simulink model "mobrob_sim"  (Simulink 7.2)
settings: Solver=ode45  StartTime=0.0  StopTime=60  FixedStep=0.1*Ts  RelTol=1e-3
values from neighbouring files (symbols this model uses):
  robot = jacobian(robot, q)    [contactforce.m]    (also in dirkin.m = robotIn; dyn.m = dynmodel2(robot,q,dq,Ftool); dynmodel.m = neinit(robotIn,q); dynmodel2.m = neinit(robotIn,q))
  x0 = 0    [RV_EKF_sim.m]    (also in dyn.m = [q0; dq0])
undefined symbols (not defined in the file or in its folder): ctrlparam, map
settings Model: Creator=Cupec  LastModifiedBy=Cupec
settings OptimizationCC: InitFltsAndDblsToZero=on
settings DebuggingCC: SaveWithParameterizedLinksMsg=none  SignalResolutionControl=TryResolveAllWithWarning  MultiTaskDSMMsg=warning  MultiTaskCondExecSysMsg=none
settings RTWCC: IncludeERTFirstTime=on
settings GRTTargetCC: TargetFcnLib=ansi_tfl_tmw.mat

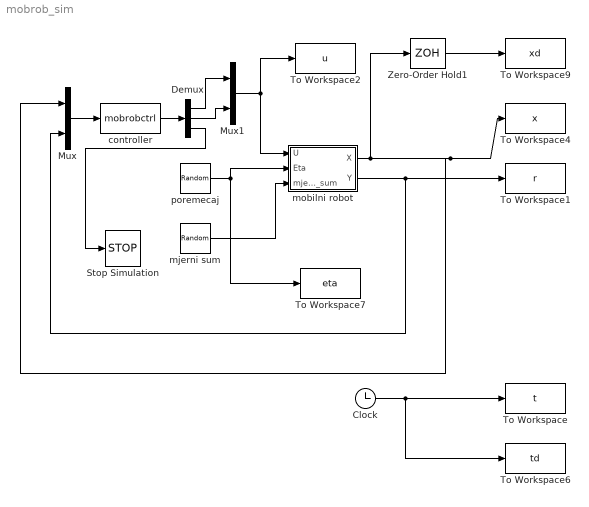
== system mobrob_sim ==
  Clock : Clock
      settings: Decimation=10
  Demux : Demux  Outputs=3
  Mux : Mux  Inputs=2
  Mux1 : Mux  Inputs=2
  Stop Simulation : Stop
  To Workspace : ToWorkspace  VariableName=t  SampleTime=-1  SaveFormat=Array
  To Workspace1 : ToWorkspace  VariableName=r  SampleTime=0.1*robot.TS  SaveFormat=Array
  To Workspace2 : ToWorkspace  VariableName=u  SampleTime=0.1*ctrlparam.T  SaveFormat=Array
  To Workspace4 : ToWorkspace  VariableName=x  SampleTime=-1  SaveFormat=Array
  To Workspace6 : ToWorkspace  VariableName=td  SampleTime=0.1*ctrlparam.T  SaveFormat=Array
  To Workspace7 : ToWorkspace  VariableName=eta  SampleTime=0.1*ctrlparam.T  SaveFormat=Array
  To Workspace9 : ToWorkspace  VariableName=xd  SampleTime=0.1*ctrlparam.T  SaveFormat=Array
  Zero-Order Hold1 : ZeroOrderHold  SampleTime=ctrlparam.T
  controller : S-Function  FunctionName=mobrobctrl  Parameters=robot,ctrlparam,map  EnableBusSupport=off
  mjerni sum : RandomNumber  Mean=zeros(robot.nS,1)  Variance=robot.varnoise*ones(robot.nS,1)  Seed=100100  SampleTime=0.1*ctrlparam.T
  mobilni robot : Subsystem
  poremecaj : RandomNumber  Mean=zeros(2,1)  Variance=robot.vardisturb*ones(2,1)  Seed=[30018 67776]'  SampleTime=0.1*ctrlparam.T
  wires:
  Clock/1 -> To Workspace/1, To Workspace6/1
  mobilni robot/1(X) -> Zero-Order Hold1/1, To Workspace4/1, Mux/1
  poremecaj/1 -> To Workspace7/1, mobilni robot/2(Eta)
  Mux/1 -> controller/1
  Zero-Order Hold1/1 -> To Workspace9/1
  mjerni sum/1 -> mobilni robot/3(mjerni_sum)
  mobilni robot/2(Y) -> To Workspace1/1, Mux/2
  controller/1 -> Demux/1
  Demux/1 -> Mux1/1
  Demux/2 -> Mux1/2
  Mux1/1 -> To Workspace2/1, mobilni robot/1(U)
  Demux/3 -> Stop Simulation/1

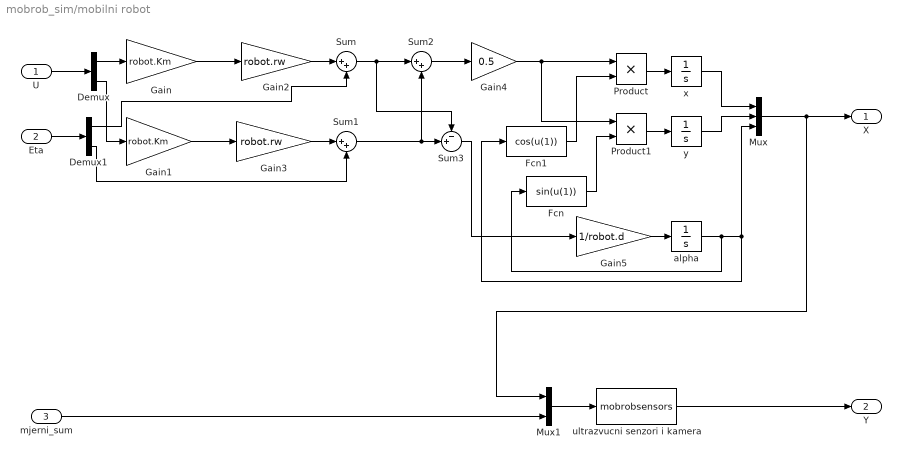
== system mobrob_sim/mobilni robot ==
  U : Inport  OutDataType=sfix(16)  OutScaling=2^0
  Eta : Inport  Port=2  OutDataType=sfix(16)  OutScaling=2^0
  mjerni_sum : Inport  Port=3  OutDataType=sfix(16)  OutScaling=2^0
  Demux : Demux  Outputs=[1 1]
  Demux1 : Demux  Outputs=[1 1]
  Fcn : Fcn  Expr=sin(u(1))
  Fcn1 : Fcn  Expr=cos(u(1))
  Gain : Gain  Gain=robot.Km  ParameterDataType=sfix(16)  ParameterScaling=2^0  OutDataType=sfix(16)  OutScaling=2^0
  Gain1 : Gain  Gain=robot.Km  ParameterDataType=sfix(16)  ParameterScaling=2^0  OutDataType=sfix(16)  OutScaling=2^0
  Gain2 : Gain  Gain=robot.rw  ParameterDataType=sfix(16)  ParameterScaling=2^0  OutDataType=sfix(16)  OutScaling=2^0
  Gain3 : Gain  Gain=robot.rw  ParameterDataType=sfix(16)  ParameterScaling=2^0  OutDataType=sfix(16)  OutScaling=2^0
  Gain4 : Gain  Gain=0.5  ParameterDataType=sfix(16)  ParameterScaling=2^0  OutDataType=sfix(16)  OutScaling=2^0
  Gain5 : Gain  Gain=1/robot.d  ParameterDataType=sfix(16)  ParameterScaling=2^0  OutDataType=sfix(16)  OutScaling=2^0
  Mux : Mux  Inputs=3
  Mux1 : Mux  Inputs=2
  Product : Product  OutDataType=sfix(16)  OutScaling=2^0  RndMeth=Zero
  Product1 : Product  OutDataType=sfix(16)  OutScaling=2^0  RndMeth=Zero
  Sum : Sum  Inputs=|++  OutDataType=sfix(16)  OutScaling=2^0
  Sum1 : Sum  Inputs=|++  OutDataType=sfix(16)  OutScaling=2^0
  Sum2 : Sum  Inputs=|++  OutDataType=sfix(16)  OutScaling=2^0
  Sum3 : Sum  Inputs=-+|  OutDataType=sfix(16)  OutScaling=2^0
  alpha : Integrator  InitialCondition=x0(3)
  ultrazvucni senzori i kamera : S-Function  FunctionName=mobrobsensors  Parameters=robot,map  EnableBusSupport=off
  x : Integrator  InitialCondition=x0(1)
  y : Integrator  InitialCondition=x0(2)
  X : Outport  OutDataType=sfix(16)  OutScaling=2^0
  Y : Outport  Port=2  OutDataType=sfix(16)  OutScaling=2^0
  wires:
  Gain/1 -> Gain2/1
  Gain1/1 -> Gain3/1
  Gain2/1 -> Sum/1
  Gain3/1 -> Sum1/1
  Sum/1 -> Sum2/1, Sum3/1
  Sum1/1 -> Sum2/2, Sum3/2
  Sum2/1 -> Gain4/1
  U/1 -> Demux/1
  Demux/1 -> Gain/1
  Demux/2 -> Gain1/1
  Eta/1 -> Demux1/1
  Demux1/1 -> Sum/2
  Demux1/2 -> Sum1/2
  Mux/1 -> X/1, Mux1/1
  x/1 -> Mux/1
  y/1 -> Mux/2
  alpha/1 -> Mux/3, Fcn1/1, Fcn/1
  Product/1 -> x/1
  Fcn1/1 -> Product/2
  Gain4/1 -> Product/1, Product1/1
  Product1/1 -> y/1
  Fcn/1 -> Product1/2
  Gain5/1 -> alpha/1
  Sum3/1 -> Gain5/1
  Mux1/1 -> ultrazvucni senzori i kamera/1
  mjerni_sum/1 -> Mux1/2
  ultrazvucni senzori i kamera/1 -> Y/1
